simulink model "SoC"  (R2022a)
settings: Solver=FixedStepAuto  StartTime=0.0  StopTime=14000  RelTol=1e-3
settings Model: Creator=dwegg  LastModifiedBy=joser
settings SolverCC: AlgebraicLoopSolver=TrustRegion
settings DataIOCC: SaveOutput=off
settings OptimizationCC: DefaultParameterBehavior=Inlined
settings DebuggingCC: UnconnectedInputMsg=warning  UnconnectedOutputMsg=warning  UnconnectedLineMsg=warning  SFMachineParentedDataDiag=warning  ArithmeticOperatorsInVariantConditions=warning
settings SFSimCC: CustomCodeUndefinedFunction=UseInterfaceOnly
settings RTWCC: Description=INTECRIO Real-Time Target  SystemTargetFile=irt.tlc  TemplateMakefile=irt_default_tmf
settings STFCustomTargetCC: TargetLangStandard=C99 (ISO)  UtilityFuncGeneration=Shared location  MatFileLogging=on  SystemTargetFile=irt.tlc
settings GRTTargetCC: UtilityFuncGeneration=Shared location  ParMdlRefBuildCompliant=off  CompOptLevelCompliant=off  ConcurrentExecutionCompliant=off  CombineOutputUpdateFcns=off  CPPClassGenCompliant=off  GRTInterface=on  UseToolchainInfoCompliant=off  GenerateASAP2=on

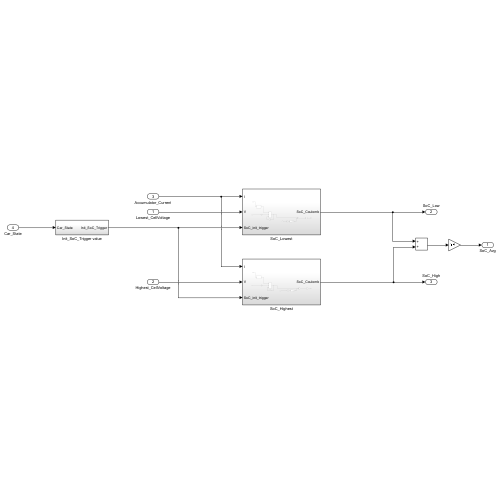
[thumbnail: Simulink's stored preview of the top-level diagram]
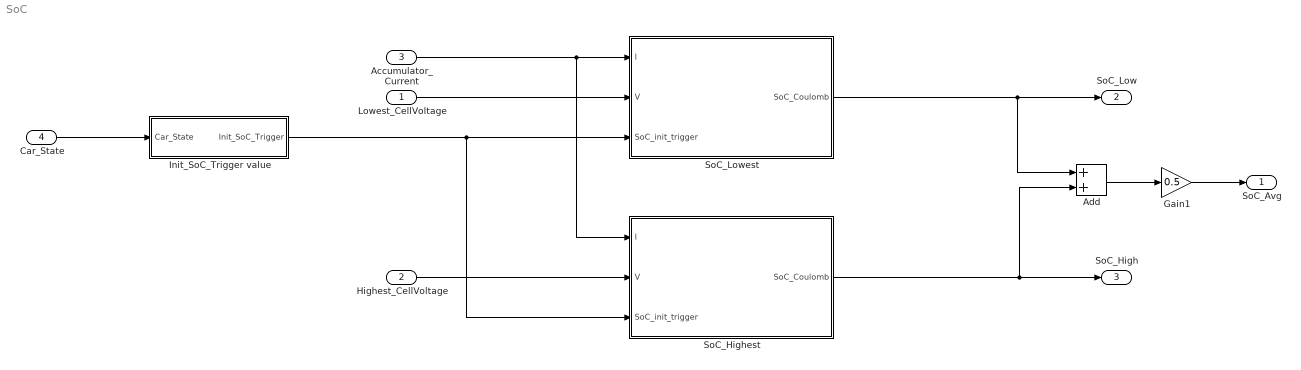
== system SoC ==
  Lowest_CellVoltage : Inport
  Highest_CellVoltage : Inport  Port=2
  Accumulator_Current : Inport  Port=3
  Car_State : Inport  Port=4
  Add : Sum
  Gain1 : Gain  Gain=0.5
  Init_SoC_Trigger value : Subsystem
  SoC_Highest : Subsystem
  SoC_Lowest : Subsystem
  SoC_Avg : Outport
  SoC_Low : Outport  Port=2
  SoC_High : Outport  Port=3
  wires:
  Lowest_CellVoltage/1 -> SoC_Lowest/2(V)
  Init_SoC_Trigger value/1(Init_SoC_Trigger) -> SoC_Highest/3(SoC_init_trigger), SoC_Lowest/3(SoC_init_trigger)
  Accumulator_Current/1 -> SoC_Highest/1(I), SoC_Lowest/1(I)
  SoC_Lowest/1(SoC_Coulomb) -> Add/1, SoC_Low/1
  SoC_Highest/1(SoC_Coulomb) -> Add/2, SoC_High/1
  Add/1 -> Gain1/1
  Gain1/1 -> SoC_Avg/1
  Highest_CellVoltage/1 -> SoC_Highest/2(V)
  Car_State/1 -> Init_SoC_Trigger value/1(Car_State)

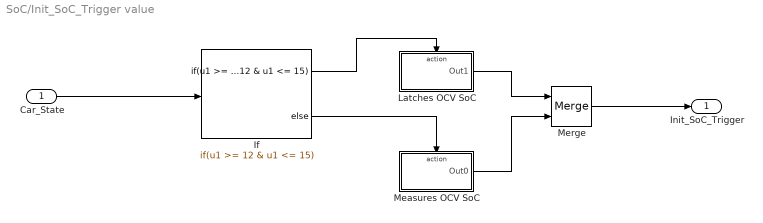
== system SoC/Init_SoC_Trigger value ==
  Car_State : Inport
  If : If  IfExpression=u1 >= 12 & u1 <= 15
  Latches OCV SoC : Subsystem  TreatAsAtomicUnit=on
  Measures OCV SoC : Subsystem  TreatAsAtomicUnit=on
  Merge : Merge
  Init_SoC_Trigger : Outport  VectorParamsAs1DForOutWhenUnconnected=off
  wires:
  Car_State/1 -> If/1
  If/1 -> Latches OCV SoC/Action
  If/2 -> Measures OCV SoC/Action
  Measures OCV SoC/1(Out0) -> Merge/2
  Latches OCV SoC/1(Out1) -> Merge/1
  Merge/1 -> Init_SoC_Trigger/1

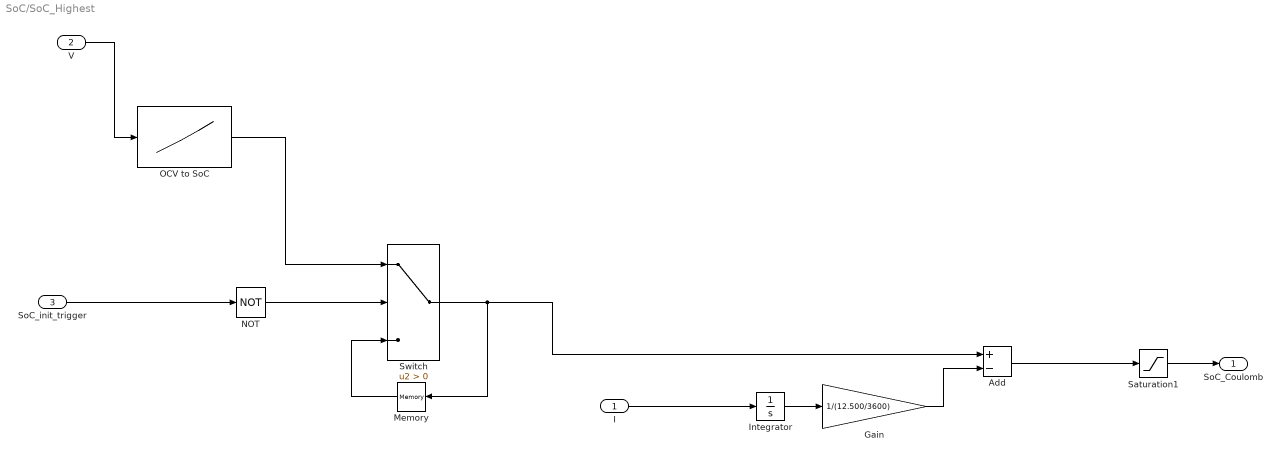
== system SoC/SoC_Highest ==
  I : Inport
  V : Inport  Port=2
  SoC_init_trigger : Inport  Port=3
  Add : Sum  Inputs=+-
  Gain : Gain  Gain=1/(12.500/3600)
  Integrator : Integrator
  Memory : Memory
  NOT : Logic  Operator=NOT  IconShape=distinctive  AllPortsSameDT=off  OutDataTypeStr=boolean
  OCV to SoC : Lookup_n-D  NumberOfTableDimensions=1  BreakpointsForDimension1=|  Table=|  InternalRulePriority=Speed  RndMeth=Simplest
      BreakpointsForDimension1=|
      | [2.94959022892031
      | 3.21416977318498
      | 3.34338141328538
      | 3.38823547157865
      | 3.42107134634789
      | 3.48650481123582
      | 3.51335866761468
      | 3.54070339538832
      | 3.56968305677313
      | 3.63185877907628
      | 3.63255716896237
      | 3.64803371545993
      | 3.66548496788278
      | 3.66563518858557
      | 3.72681148156897
      | 3.76406010705888
      | 3.77075982343748
      | 3.84270466053206
      | 3.84295206305238
      | 3.90164564850831
      | 3.96498508551296
      | 3.96615700649565
      | 4.04797311953080
      | 4.07602027520885
      | 4.10936207844059
      | 4.18278376875771]
      Table=|
      | [0.00364887820512694
      | 0.0406322115384605
      | 0.0806891025641018
      | 0.120744391025641
      | 0.160802083333333
      | 0.200854967948718
      | 0.240911057692307
      | 0.280964743589743
      | 0.321025641025641
      | 0.361079326923077
      | 0.401137019230769
      | 0.441193910256410
      | 0.481247596153846
      | 0.521301282051282
      | 0.561357371794872
      | 0.601413461538462
      | 0.641456730769231
      | 0.681509615384616
      | 0.721566506410257
      | 0.761620993589744
      | 0.801677884615385
      | 0.841734775641026
      | 0.881788461538462
      | 0.921837339743590
      | 0.961899038461539
      | 0.998685256410256]
  Saturation1 : Saturate  UpperLimit=100  LowerLimit=0
  Switch : Switch  Criteria=u2 > Threshold  ZeroCross=off  SaturateOnIntegerOverflow=off  InputSameDT=off
  SoC_Coulomb : Outport  VectorParamsAs1DForOutWhenUnconnected=off
  wires:
  Saturation1/1 -> SoC_Coulomb/1
  SoC_init_trigger/1 -> NOT/1
  NOT/1 -> Switch/2
  Memory/1 -> Switch/3
  OCV to SoC/1 -> Switch/1
  V/1 -> OCV to SoC/1
  Add/1 -> Saturation1/1
  Integrator/1 -> Gain/1
  I/1 -> Integrator/1
  Switch/1 -> Add/1, Memory/1
  Gain/1 -> Add/2

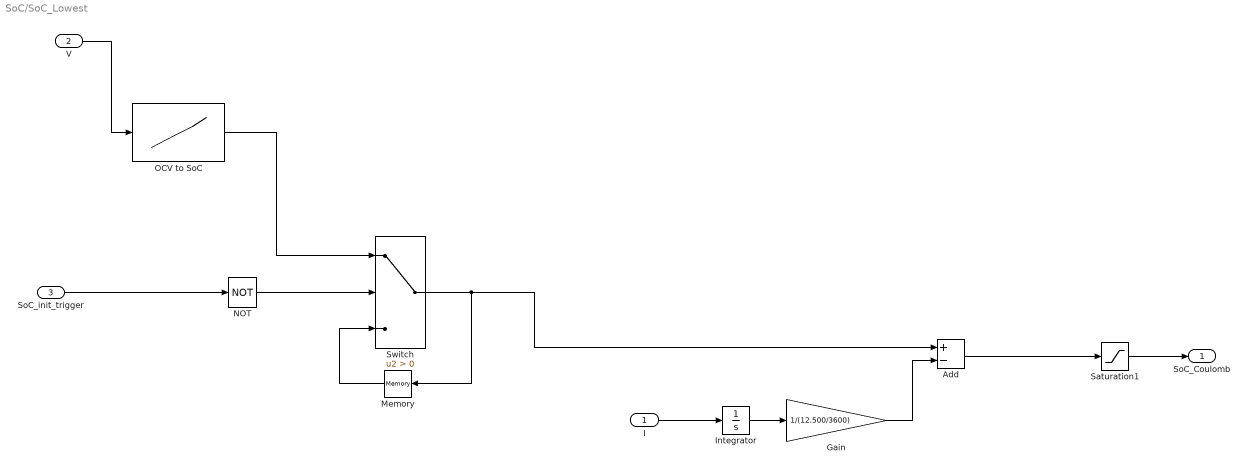
== system SoC/SoC_Lowest ==
  I : Inport
  V : Inport  Port=2
  SoC_init_trigger : Inport  Port=3
  Add : Sum  Inputs=+-
  Gain : Gain  Gain=1/(12.500/3600)
  Integrator : Integrator
  Memory : Memory
  NOT : Logic  Operator=NOT  IconShape=distinctive  AllPortsSameDT=off  OutDataTypeStr=boolean
  OCV to SoC : Lookup_n-D  NumberOfTableDimensions=1  BreakpointsForDimension1=|  Table=|  InternalRulePriority=Speed  RndMeth=Simplest
      BreakpointsForDimension1=|
      | [2.94959022892031
      | 3.21416977318498
      | 3.34338141328538
      | 3.38823547157865
      | 3.42107134634789
      | 3.48650481123582
      | 3.51335866761468
      | 3.54070339538832
      | 3.56968305677313
      | 3.63185877907628
      | 3.63255716896237
      | 3.64803371545993
      | 3.66548496788278
      | 3.66563518858557
      | 3.72681148156897
      | 3.76406010705888
      | 3.77075982343748
      | 3.84270466053206
      | 3.84295206305238
      | 3.90164564850831
      | 3.96498508551296
      | 3.96615700649565
      | 4.04797311953080
      | 4.07602027520885
      | 4.10936207844059
      | 4.18278376875771]
      Table=|
      | [0.00364887820512694
      | 0.0406322115384605
      | 0.0806891025641018
      | 0.120744391025641
      | 0.160802083333333
      | 0.200854967948718
      | 0.240911057692307
      | 0.280964743589743
      | 0.321025641025641
      | 0.361079326923077
      | 0.401137019230769
      | 0.441193910256410
      | 0.481247596153846
      | 0.521301282051282
      | 0.561357371794872
      | 0.601413461538462
      | 0.641456730769231
      | 0.681509615384616
      | 0.721566506410257
      | 0.761620993589744
      | 0.801677884615385
      | 0.841734775641026
      | 0.881788461538462
      | 0.921837339743590
      | 0.961899038461539
      | 0.998685256410256]
  Saturation1 : Saturate  UpperLimit=100  LowerLimit=0
  Switch : Switch  Criteria=u2 > Threshold  ZeroCross=off  SaturateOnIntegerOverflow=off  InputSameDT=off
  SoC_Coulomb : Outport  VectorParamsAs1DForOutWhenUnconnected=off
  wires:
  Add/1 -> Saturation1/1
  I/1 -> Integrator/1
  Switch/1 -> Memory/1, Add/1
  V/1 -> OCV to SoC/1
  OCV to SoC/1 -> Switch/1
  Memory/1 -> Switch/3
  NOT/1 -> Switch/2
  SoC_init_trigger/1 -> NOT/1
  Saturation1/1 -> SoC_Coulomb/1
  Integrator/1 -> Gain/1
  Gain/1 -> Add/2

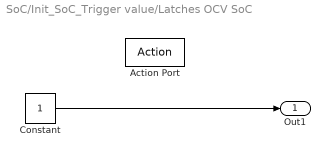
== system SoC/Init_SoC_Trigger value/Latches OCV SoC ==
  Action Port : ActionPort  ActionPortLabel=if(u1 >= 12 & u1 <= 15)
  Constant : Constant
  Out1 : Outport  VectorParamsAs1DForOutWhenUnconnected=off
  wires:
  Constant/1 -> Out1/1

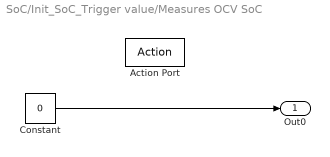
== system SoC/Init_SoC_Trigger value/Measures OCV SoC ==
  Action Port : ActionPort  ActionPortLabel=else
  Constant : Constant  Value=0
  Out0 : Outport  VectorParamsAs1DForOutWhenUnconnected=off
  wires:
  Constant/1 -> Out0/1
